simulink model "essais_1"  (R2019a)
settings: Solver=VariableStepAuto  StartTime=0.0  StopTime=10.0  RelTol=1e-3
undefined symbols (not defined in the file): sigbuilder_block
libraries: vehdynlibtire x4, vehdynlibsuspension x1, vehdynlibeom x1
(part 2 of 2)

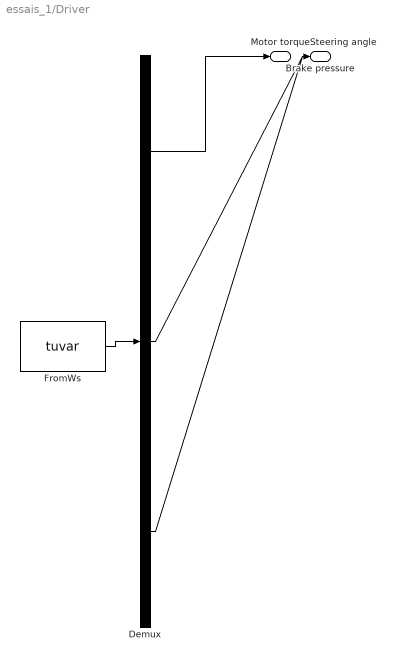
== system essais_1/Driver  ==
  Demux : Demux  Tag=STV Demux  Outputs=3
  FromWs : FromWorkspace  Tag=STV FromWs  VariableName=tuvar  SampleTime=0
      SigBuilderData=|
      | common.afterFinalStr = 'Extrapolate'
      | common.sampleTime = 0
      | dataSet.timeRange = [0 10]
      | dataSet.name = 'Group 1'
      | sbobj.Groups.Name = 'Group 1'
      | sbobj.Groups.Signals(1).Name = 'Motor torque'
      | sbobj.Groups.Signals(1).XData = [0 1 1 6 6 10]
      | sbobj.Groups.Signals(1).YData = [0 0 1 1 0 0]
      | sbobj.Groups.Signals(2).Name = 'Brake pressure'
      | sbobj.Groups.Signals(2).XData = [0 10]
      | sbobj.Groups.Signals(2).YData = [0 0]
      | sbobj.Groups.Signals(3).Name = 'Steering angle'
      | sbobj.Groups.Signals(3).XData = [0 10]
      | sbobj.Groups.Signals(3).YData = [0 0]
  Motor torque : Outport  Tag=STV Outport
  Brake pressure : Outport  Tag=STV Outport  Port=2
  Steering angle : Outport  Tag=STV Outport  Port=3
  wires:
  Demux/1 -> Motor torque/1
  FromWs/1 -> Demux/1
  Demux/2 -> Brake pressure/1
  Demux/3 -> Steering angle/1
